simulink model "Kalman_EMPhase_Simulink"  (R2019b)
settings: Solver=VariableStepAuto  StartTime=0.0  StopTime=model.sim_dur  FixedStep=0.01  RelTol=1e-3
undefined symbols (not defined in the file or in its folder): Discrete, model, Time
libraries: dspsrcs4 x4, ctrlSharedLib x2
settings Model: Creator=isidoraradenkovic  LastModifiedBy=isidoraradenkovic
settings DataIOCC: ReturnWorkspaceOutputs=off
settings OptimizationCC: DefaultParameterBehavior=Inlined  PassReuseOutputArgsAs=Individual arguments  EfficientTunableParamExpr=on
settings DebuggingCC: ParameterTunabilityLossMsg=error  ArithmeticOperatorsInVariantConditions=warning
settings SFSimCC: SimUseLocalCustomCode=off  MATLABDynamicMemAlloc=off  CustomCodeUndefinedFunction=UseInterfaceOnly
settings RTWCC: SystemTargetFile=ert.tlc  TemplateMakefile=ert_default_tmf  GenerateReport=on  RTWUseLocalCustomCode=off  IncludeHyperlinkInReport=on  LaunchReport=on  GenerateTraceInfo=on  GenerateTraceReport=on  GenerateTraceReportSl=on  GenerateTraceReportSf=on  GenerateTraceReportEml=on  CheckMdlBeforeBuild=Warning
settings CodeAppCC: GenerateComments=off  IgnoreCustomStorageClasses=off  SimulinkBlockComments=off
settings ERTTargetCC: TargetLangStandard=C99 (ISO)  GenerateSampleERTMain=on  InlinedParameterPlacement=NonHierarchical  ERTCustomFileTemplate=example_file_process.tlc
settings SimscapeCC: SimscapeNormalizeSystem=off

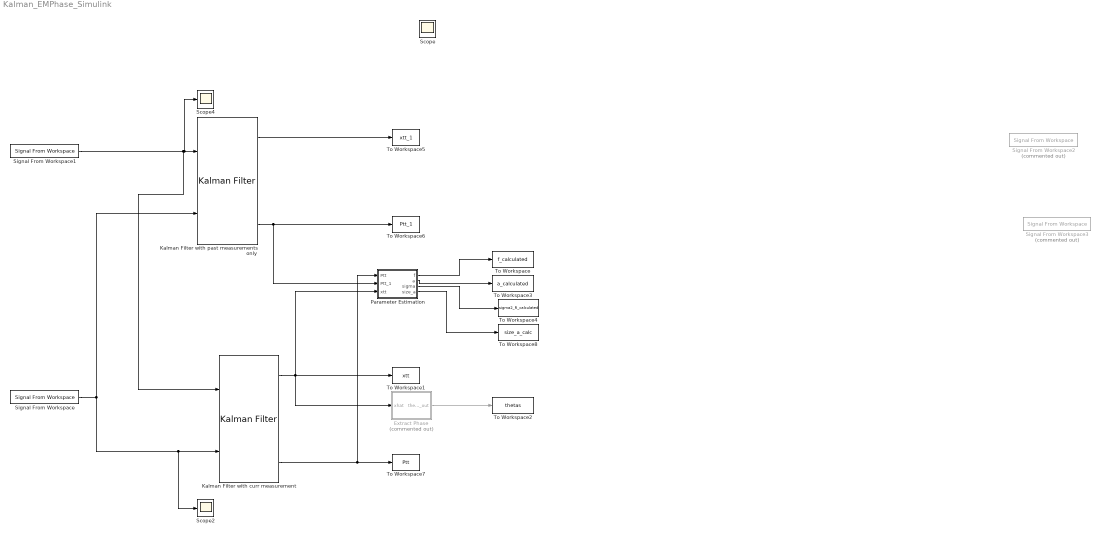
== system Kalman_EMPhase_Simulink ==
  Extract Phase : MATLAB Function  Commented=on  TreatAsAtomicUnit=on  SystemSampleTime=model.Ts
  Kalman Filter with curr measurement : ctrlSharedLib/Kalman Filter  TimeDomain=Discrete-Time  UseCurrentEstimator=on  ModelSource=Individual A, B, C, D matrices  ModelSourceVariable=ss(0.95,1,1,0,1)  A=model.A  B=model.B  C=model.C  D=0  NumberOfStates=1  NumberOfInputs=1  NumberOfOutputs=1  InitialEstimateSource=Dialog  X0=model.x_0  P0=Q_const  UseK=off  UseGH=on  NumberOfProcessNoiseInputs=1  G=model.Gm  TimeInvariantG=on  H=0  TimeInvariantH=on  Q=model.Q  TimeInvariantQ=on  R=model.R  TimeInvariantR=on  N=0  TimeInvariantN=on  AddInputPort=on  AddEnablePort=off  OutputEstimatedY=on  OutputP=on  Ts=model.Ts
      settings: SourceProductBaseCode=CT
  Kalman Filter with past measurements only : ctrlSharedLib/Kalman Filter  TimeDomain=Discrete-Time  UseCurrentEstimator=off  ModelSource=Individual A, B, C, D matrices  ModelSourceVariable=ss(0.95,1,1,0,1)  A=model.A  B=model.B  C=model.C  D=0  NumberOfStates=1  NumberOfInputs=1  NumberOfOutputs=1  InitialEstimateSource=Dialog  X0=model.x_0  P0=Q_const  UseK=off  UseGH=on  NumberOfProcessNoiseInputs=1  G=model.Gm  TimeInvariantG=on  H=0  TimeInvariantH=on  Q=model.Q  TimeInvariantQ=on  R=model.R  TimeInvariantR=on  N=0  TimeInvariantN=on  AddInputPort=on  AddEnablePort=off  OutputEstimatedY=on  OutputP=on  Ts=model.Ts
      settings: SourceProductBaseCode=CT
  Parameter Estimation : MATLAB Function  TreatAsAtomicUnit=on  SystemSampleTime=model.Ts
  Scope2 : Scope
  Scope4 : Scope
  Signal From Workspace : dspsrcs4/Signal From Workspace  X=input_data  Ts=model.Ts  nsamps=1  OutputAfterFinalValue=Cyclic repetition  ignoreOrWarnInputAndFrameLengths=off  OutputFrames=off
  Signal From Workspace1 : dspsrcs4/Signal From Workspace  X=tms_pulses  Ts=model.Ts  nsamps=1  OutputAfterFinalValue=Cyclic repetition  ignoreOrWarnInputAndFrameLengths=off  OutputFrames=off
  Signal From Workspace2 : dspsrcs4/Signal From Workspace  Commented=on  X=model.Q  Ts=model.Ts  nsamps=1  OutputAfterFinalValue=Cyclic repetition  ignoreOrWarnInputAndFrameLengths=off  OutputFrames=off
  Signal From Workspace3 : dspsrcs4/Signal From Workspace  Commented=on  X=model.R  Ts=model.Ts  nsamps=1  OutputAfterFinalValue=Cyclic repetition  ignoreOrWarnInputAndFrameLengths=off  OutputFrames=off
  To Workspace : ToWorkspace  VariableName=f_calculated  SampleTime=model.Ts
      settings: Save2DSignal=2-D array (concatenate along first dimension)
  To Workspace1 : ToWorkspace  VariableName=xtt  SampleTime=model.Ts
      settings: Save2DSignal=2-D array (concatenate along first dimension)
  To Workspace2 : ToWorkspace  VariableName=thetas  SampleTime=model.Ts
      settings: Save2DSignal=2-D array (concatenate along first dimension)
  To Workspace3 : ToWorkspace  VariableName=a_calculated  SampleTime=model.Ts
      settings: Save2DSignal=2-D array (concatenate along first dimension)
  To Workspace4 : ToWorkspace  VariableName=sigma2_R_calculated  SampleTime=model.Ts
      settings: Save2DSignal=2-D array (concatenate along first dimension)
  To Workspace5 : ToWorkspace  VariableName=xtt_1  SampleTime=model.Ts
      settings: Save2DSignal=2-D array (concatenate along first dimension)
  To Workspace6 : ToWorkspace  VariableName=Ptt_1  SampleTime=model.Ts
      settings: Save2DSignal=2-D array (concatenate along first dimension)
  To Workspace7 : ToWorkspace  VariableName=Ptt  SampleTime=model.Ts
      settings: Save2DSignal=2-D array (concatenate along first dimension)
  To Workspace8 : ToWorkspace  VariableName=size_a_calc  SampleTime=model.Ts
      settings: Save2DSignal=2-D array (concatenate along first dimension)
  Scope : Scope
  wires:
  Signal From Workspace/1 -> Kalman Filter with curr measurement/2, Scope2/1, Kalman Filter with past measurements only/2
  Kalman Filter with past measurements only/3 -> Parameter Estimation/2(Ptt_1), To Workspace6/1
  Kalman Filter with curr measurement/3 -> Parameter Estimation/1(Ptt), To Workspace7/1
  Signal From Workspace1/1 -> Scope4/1, Kalman Filter with past measurements only/1, Kalman Filter with curr measurement/1
  Extract Phase/1(thetas_out) -> To Workspace2/1
  Parameter Estimation/3(sigma) -> To Workspace4/1
  Parameter Estimation/2(a) -> To Workspace3/1
  Parameter Estimation/1(f) -> To Workspace/1
  Kalman Filter with curr measurement/1 -> To Workspace1/1, Parameter Estimation/3(xtt), Extract Phase/1(xhat)
  Kalman Filter with past measurements only/1 -> To Workspace5/1
  Parameter Estimation/4(size_a) -> To Workspace8/1

== matlab function Kalman_EMPhase_Simulink/Parameter Estimation ==
  data: Ptt input; f output size=model.num_rhythms; Ptt_1 input; xtt input; a output size=[2*model.num_rhythms, 2*model.num_rhythms]; sigma output size=[2*model.num_rhythms, 2*model.num_rhythms]; model parameter; size_a output size=2
function [f, a, sigma, size_a]  = parameter_estimation(Ptt, Ptt_1, xtt, model)

if length(xtt) == (model.param_est_length+2)*(2*model.num_rhythms)
    %%Backward Smoothing
    [PttN, xttN, Ptt_1N, xforwN, PforwN] = backward_smoothing(model, Ptt, Ptt_1, xtt);
    
    %%EM parameter estimation
    [f, a, sigma, size_a]  = em_method(model, PttN, xttN, Ptt_1N, xforwN, PforwN);
else
    f = model.f;
    a = model.a;
    sigma = model.sigma2_R; %CORRECT
    size_a = [77; 88];
end


end

function [PttN, xttN, Ptt_1N, xforwN, PforwN] = backward_smoothing(model, Ptt, Ptt_1, xtt)
dimensions = model.state_dimensions;
length = model.param_est_length;

PttN = zeros(dimensions * length, dimensions); % For the smoothing step
xttN = zeros(length, dimensions);
Ptt_1N = zeros(dimensions * length, dimensions); % Covariance

coder.varsize('xforwN');
coder.varsize('PforwN');
xforwN = xtt(length+1, :);
PforwN = Ptt((dimensions * length+1):(dimensions * (length+1)), :);


for j= (length+1):(-1):2 % The paper is 0 indexed, MATLAB is 1 indexed
    % Extract matrices for simpler representation
    % Index (j-1) becomes:
    % ((j-2)*dimensions+1):((j-1)*dimensions)
    % Index j becomes:
    % ((j-1)*dimensions+1):(j*dimensions)
    ind_prev = ((j-2)*dimensions+1):((j-1)*dimensions);
    ind_curr = ((j-1)*dimensions+1):(j*dimensions);
    Pt_1_prev = Ptt_1(ind_prev, :);
    Pt_1_curr = Ptt_1(ind_curr, :);
    Pt_prev = Ptt(ind_prev, :);
    %xt_prev = xtt(j-1, :);
    xt_prev = xtt(j-1, 1:2);
    
    J = Pt_1_prev\Pt_prev*model.A'; %UNSTABLE INVERSES?
    xttN(j-1, 1:dimensions) = xt_prev+(xforwN-xt_prev*(model.A'))*(J');
    PttN(ind_prev, 1:dimensions) = Pt_prev+J*(PforwN-Pt_1_curr)*J';
    %covariance is symmetric, so Ptt_1N = Pt_1tN = J*PttN hence:
    Ptt_1N(ind_prev, 1:dimensions) = J*PforwN;
    
    xforwN = xttN(j-1, :);
    PforwN = PttN(ind_prev, :);
end

end

function [f, a, sigma, size_a]  = em_method(model, PttN, xttN, Ptt_1N, xforwN, PforwN)
dimensions = model.state_dimensions;
l = model.param_est_length;
num_rhythms = model.num_rhythms;

P_A = matrix_sum(PttN, dimensions);
P_B = matrix_sum(Ptt_1N, dimensions);
P_C = matrix_sum([PttN((dimensions+1):end, :); PforwN], dimensions);

xtN = [xttN(2:l, :); xforwN];
x_A_prod = matrix_product(xttN, xttN, dimensions);
x_A = matrix_sum(x_A_prod, dimensions);
x_B_prod = matrix_product(xtN, xttN, dimensions);
x_B = matrix_sum(x_B_prod, dimensions);
x_C_prod = matrix_product(xtN, xtN, dimensions);
x_C = matrix_sum(x_C_prod, dimensions);

A_smooth = P_A+x_A;
B_smooth = P_B+x_B;
C_smooth = P_C+x_C;

f = atan(rt(B_smooth, num_rhythms)./tr(B_smooth, num_rhythms));
a = sqrt(rt(B_smooth, num_rhythms).^2+tr(B_smooth, num_rhythms).^2)./tr(A_smooth, num_rhythms);
size_temp = size(a);
sigma = (tr(C_smooth, num_rhythms)-a.^2.*tr(A_smooth, num_rhythms))/(2*l);

f = f(model.num_rhythms);
a = a(1:2*model.num_rhythms, 1:2*model.num_rhythms); %CORRECT
sigma = sigma(1:2, 1:2);
size_a = size_temp(1:2)';
end

== matlab function Kalman_EMPhase_Simulink/Extract Phase ==
  data: xhat input; thetas_out output
function thetas_out  = extract_phase(xhat)
num_rhythms = length(xhat)/2;
% thetas_out = zeros(num_rhythms, 1);
% 
% for j = 1:num_rhythms
%     Im = xhat(2 * (j-1) + 2);
%     Re = xhat(2 * (j-1) + 1);
%     thetas_out(j, 1) = atan2(Im, Re);
% end

thetas_out = atan2(xhat(2:2:2*num_rhythms), xhat(1:2:2*(num_rhythms-1)+1))
